simulink model "Qrotor"  (R2021a)
settings: Solver=VariableStepAuto  StartTime=0.0  StopTime=10.0  RelTol=1e-3
settings Model: Creator=Sirius  LastModifiedBy=Sirius

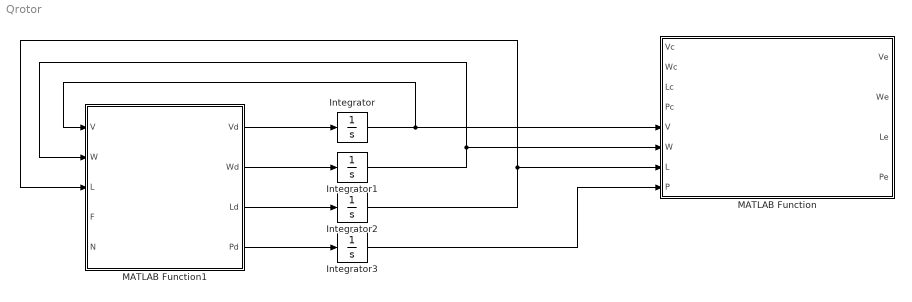
== system Qrotor ==
  Integrator{,1..3} (4 alike) : Integrator  InitialCondition=[0,0,0]  ContinuousStateAttributes='V'
  MATLAB Function : MATLAB Function  TreatAsAtomicUnit=on
  MATLAB Function1 : MATLAB Function  TreatAsAtomicUnit=on
  wires:
  MATLAB Function1/1(Vd) -> Integrator/1
  Integrator/1 -> MATLAB Function1/1(V), MATLAB Function/5(V)
  MATLAB Function1/2(Wd) -> Integrator1/1
  Integrator1/1 -> MATLAB Function1/2(W), MATLAB Function/6(W)
  MATLAB Function1/3(Ld) -> Integrator2/1
  MATLAB Function1/4(Pd) -> Integrator3/1
  Integrator2/1 -> MATLAB Function1/3(L), MATLAB Function/7(L)
  Integrator3/1 -> MATLAB Function/8(P)

== matlab function Qrotor/MATLAB Function1 ==
  data: V input; Vd output; W input; L input; F input; N input; Wd output; Ld output; Pd output
function [Vd,Wd,Ld,Pd] = QRotor(V,W,L,F,N)
%define the mass m, and the inrttia matrix J
m=1;%Kg
J=eye(3,3);
Jinv=J^-1;
Vd=-Skew(W)*V+1/m*F;
Wd=Jinv*Skew(W)*J*W+Jinv*N;
Pd=RPY2Rmat(L)*V;
Ld=RPY2Qmat(L)*W;
end

== matlab function Qrotor/MATLAB Function ==
  data: Vc input; Wc input; Lc input; Ve output; We output; Le output; Pc input; V input; W input; L input; Pe output; P input
function [Ve,We,Le,Pe] = NLT(Vc,Wc,Lc,Pc,V,W,L,P)
R=RPY2Rmat(L);
Rt=R';
Rc=RPY2Rmat(Lc);


Ve=V-Vc;
We=W-Wc;
Pe=Rt*(P-Pc);
%Rc:C->I
%R:B->I
Le=Rmat2PRY(Rc'*R);
